simulink model "RotaryPendulum_SLdemo"  (R2016b)
settings: Solver=ode45  StartTime=0.0  StopTime=20  RelTol=1e-13  EnableMultiTasking=on
libraries: vrlib x1, aerolibanimutils x1
settings Model: Creator=mischak  LastModifiedBy=mischak
settings DataIOCC: LimitDataPoints=on  SaveFormat=Array
settings OptimizationCC: LifeSpan=inf
settings DebuggingCC: SolverPrmCheckMsg=warning  SFUnexpectedBacktrackingDiag=warning  SFNoUnconditionalDefaultTransitionDiag=warning  SFExecutionAtInitializationDiag=none
settings HardwareCC: ProdBitPerPointer=32  ProdBitPerSizeT=32  ProdBitPerPtrDiffT=32  ProdLargestAtomicFloat=None  ProdIntDivRoundTo=Undefined  ProdEndianess=Unspecified  ProdWordSize=32  ProdHWDeviceType=32-bit Generic
settings ModelReferenceCC: PropagateSignalLabelsOutOfModel=off
settings GRTTargetCC: TargetLangStandard=C89/C90 (ANSI)  GeneratePreprocessorConditionals=Disable all
settings ConfigComp: CovMetricSettings=dw  CovHtmlReporting=on  CovSaveCumulativeToWorkspaceVar=on  CovSaveSingleToWorkspaceVar=on  CovExternalEMLEnable=off  CovSFcnEnable=off

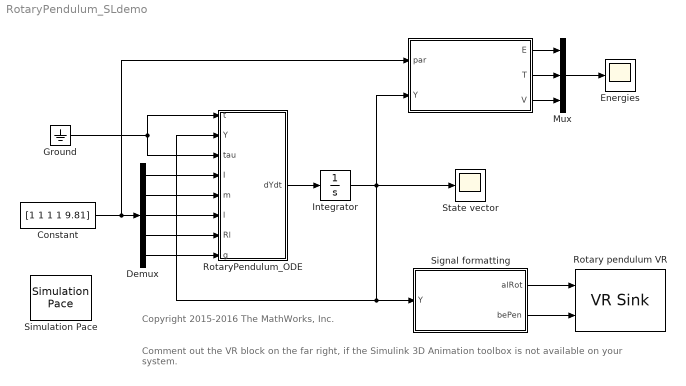
== system RotaryPendulum_SLdemo ==
  note: Comment out the VR block on the far right, if the Simulink 3D Animation toolbox is not available on your system.
  note: Copyright 2015-2016 The MathWorks, Inc.
  " " : MATLAB Function  TreatAsAtomicUnit=on
  Constant : Constant  Value=[1 1 1 1 9.81]
  Demux : Demux  Outputs=5
  Energies : Scope
  Ground : Ground
  Integrator : Integrator  InitialCondition=[0 0 0.1 0]
  Mux : Mux  Inputs=3
  Rotary pendulum VR : vrlib/VR Sink  InstantiateOnLoad=on  SampleTime=-1  ViewEnable=on  RemoteChange=off  RemoteView=off  FieldsWritten=RotaryArm.rotation.4.1.1.double#Pendulum.rotation.4.1.1.double  WorldFileName=RotaryPendulum_VR.WRL  AutoView=on  VideoDimensions=[]  AllowVariableSize=off  FigureProperties="{'Position', 'Name', 'Viewpoint', 'CameraBound', 'CameraDirection', 'CameraPosition', 'CameraUpVector', 'ZoomFactor', 'Antialiasing', 'Headlight', 'Lighting', 'NavPanel', 'Sound', 'StatusBar', 'Stereo3D', 'Stereo3DCameraOffset', 'Stereo3DHIT', 'ToolBar', 'Textures', 'Transparency', 'Triad', 'Wireframe', 'NavZones', 'NavMode', 'NavSpeed', 'CaptureFileFormat', 'CaptureFileName', 'Record2DCompressMethod', 'Record2DCompressQuality', 'Record2D', 'Record2DFileName', 'Record2DFPS'; [2.2436633663366339e+02   1.0070297029702965e+02   5.7695049504950498e+02   3.9958415841584167e+02], '', '', 'on', [0.0000000000000000e+00   0.0000000000000000e+00  -1.0000000000000000e+00], [0.0000000000000000e+00   0.0000000000000000e+00   1.0000000000000000e+01], [0.0000000000000000e+00   1.0000000000000000e+00   0.0000000000000000e+00], [1.0000000000000000e+00], 'on', 'on', 'on', 'halfbar', 'on', 'on', 'off', [1.0000000149011612e-01], [0.0000000000000000e+00], 'on', 'on', 'on', 'none', 'off', 'off', 'fly', 'normal', 'tif', '%f_anim_%n.tif', 'auto', [7.5000000000000000e+01], 'off', '%f_anim_%n.avi', 'auto'}"  mask(Virtual Reality Sink){}
      mask Display: image(imread('RotaryPendulum_icon.png'))
  RotaryPendulum_ODE : MATLAB Function  TreatAsAtomicUnit=on
  Signal formatting : MATLAB Function  TreatAsAtomicUnit=on
  Simulation Pace : aerolibanimutils/Simulation Pace  SimulationPace=1  SleepMode=MATLAB Thread  OutputPaceError=off  SampleTime=1/30
      settings: AttributesFormatString=%<SimulationPace> sec/sec
  State vector : Scope
  wires:
  Integrator/1 -> RotaryPendulum_ODE/2(Y), Signal formatting/1(Y), " "/2(Y), State vector/1
  Demux/1 -> RotaryPendulum_ODE/4(I)
  Demux/3 -> RotaryPendulum_ODE/6(l)
  Demux/4 -> RotaryPendulum_ODE/7(Rl)
  Demux/5 -> RotaryPendulum_ODE/8(g)
  Constant/1 -> " "/1(par), Demux/1
  Ground/1 -> RotaryPendulum_ODE/1(t), RotaryPendulum_ODE/3(tau)
  Signal formatting/1(alRot) -> Rotary pendulum VR/1
  Signal formatting/2(bePen) -> Rotary pendulum VR/2
  " "/2(T) -> Mux/2
  " "/1(E) -> Mux/1
  " "/3(V) -> Mux/3
  Mux/1 -> Energies/1
  Demux/2 -> RotaryPendulum_ODE/5(m)
  RotaryPendulum_ODE/1(dYdt) -> Integrator/1

== matlab function RotaryPendulum_SLdemo/  ==
  data: par input; Y input; E output; T output; V output
function [E,T,V] = ComputeEnergies(par,Y)
%#codegen
al  = Y(1);
dal = Y(2);
be  = Y(3);
dbe = Y(4);

I   = par(1);
m   = par(2);
l   = par(3);
R   = par(4);
g   = par(5);

T   = I*dal.^2/2 + m/2*(R^2*dal.^2 + l^2*dal.^2.*sin(be).^2/3 + ...
        l^2*dbe.^2/4 - R*l*dal.*dbe.*cos(be)) + m*l^2*dbe.^2/24;
V   = m*g*l/2*cos(be);
E   = T + V;
end

== matlab function RotaryPendulum_SLdemo/Signal formatting ==
  data: alRot output; bePen output; Y input
function [alRot, bePen] = FormatOUT(Y)
al    = Y(1);
dal   = Y(2);
be    = Y(3);
dbe   = Y(4);

alRot = [0; 1; 0; al];
bePen = [0; 0; 1; be];
end

== matlab function RotaryPendulum_SLdemo/RotaryPendulum_ODE ==
  data: t input; dYdt output; Y input; tau input; I input; m input; l input; Rl input; g input
function dYdt = RotaryPendulum_ODE(t,Y,tau,I,m,l,Rl,g)
%#codegen

%    This function was generated by the Symbolic Math Toolbox version 7.1.
%    19-Oct-2016 14:08:13

t4 = Y(3);
t2 = sin(t4);
t3 = Rl.^2;
t5 = cos(t4);
t6 = Y(4);
t7 = t5.^2;
t8 = Y(2);
t9 = l.^2;
t10 = I.*1.2e1;
t11 = m.*t3.*1.2e1;
t12 = t2.^2;
t13 = m.*t9.*t12.*4.0;
t14 = t10+t11+t13-m.*t3.*t7.*9.0;
t15 = 1.0./t14;
t16 = t8.^2;
t17 = t6.^2;
dYdt = [t8;t15.*(tau.*1.2e1+Rl.*g.*m.*t2.*t5.*9.0-Rl.*l.*m.*t2.*t17.*6.0-m.*t2.*t5.*t6.*t8.*t9.*8.0+Rl.*l.*m.*t2.*t7.*t16.*6.0);t6;(t15.*(I.*g.*t2.*1.8e1+Rl.*t5.*tau.*1.8e1+g.*m.*t2.*t3.*1.8e1+I.*l.*t2.*t5.*t16.*1.2e1+g.*m.*t2.*t9.*t12.*6.0+l.*m.*t2.*t3.*t5.*t16.*1.2e1-l.*m.*t2.*t3.*t5.*t17.*9.0-Rl.*m.*t2.*t6.*t7.*t8.*t9.*1.2e1+l.*m.*t2.*t5.*t9.*t12.*t16.*4.0))./l];
